simulink model "hw3"  (R2018b)
settings: Solver=ode4  StartTime=0.0  StopTime=15  FixedStep=0.001  RelTol=1e-3
values from neighbouring files (symbols this model uses):
  H = ss(sys)    [hw3.m]
  ini = [0 0 e_0]./H.C(3)    [hw3.m]
  K = 70    [hw3.m]
settings Model: Creator=user  LastModifiedBy=user

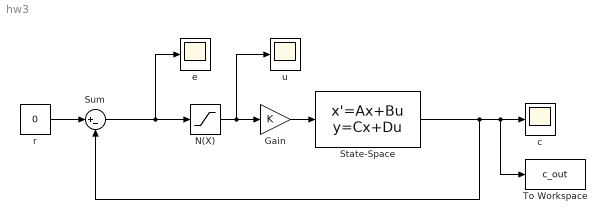
== system hw3 ==
  Gain : Gain  Gain=K
  N(X) : Saturate  UpperLimit=20  LowerLimit=-20
  State-Space : StateSpace  A=H.A  B=H.B  C=H.C  D=H.D  InitialCondition=ini
  Sum : Sum  Inputs=|+-
  To Workspace : ToWorkspace  VariableName=c_out  SaveFormat=Timeseries  SampleTime=-1
  c : Scope
  e : Scope
  r : Constant  Value=0
  u : Scope
  wires:
  State-Space/1 -> Sum/2, To Workspace/1, c/1
  N(X)/1 -> u/1, Gain/1
  r/1 -> Sum/1
  Sum/1 -> e/1, N(X)/1
  Gain/1 -> State-Space/1
